simulink model "weightloss"  (R2022a)
settings: Solver=VariableStepAuto  StartTime=0.0  StopTime=500  RelTol=1e-3
libraries: cstblocks x1
settings Model: Creator=anthony  LastModifiedBy=anthony

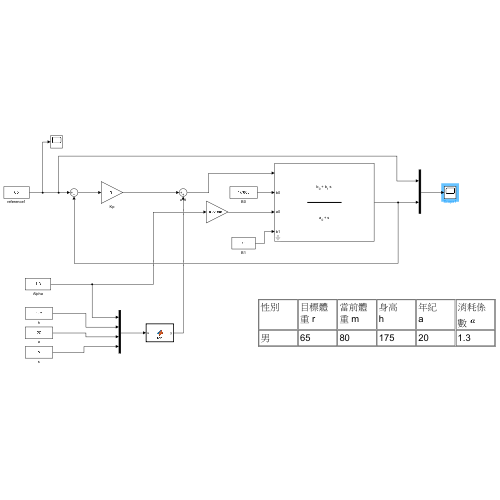
[thumbnail: Simulink's stored preview of the top-level diagram]
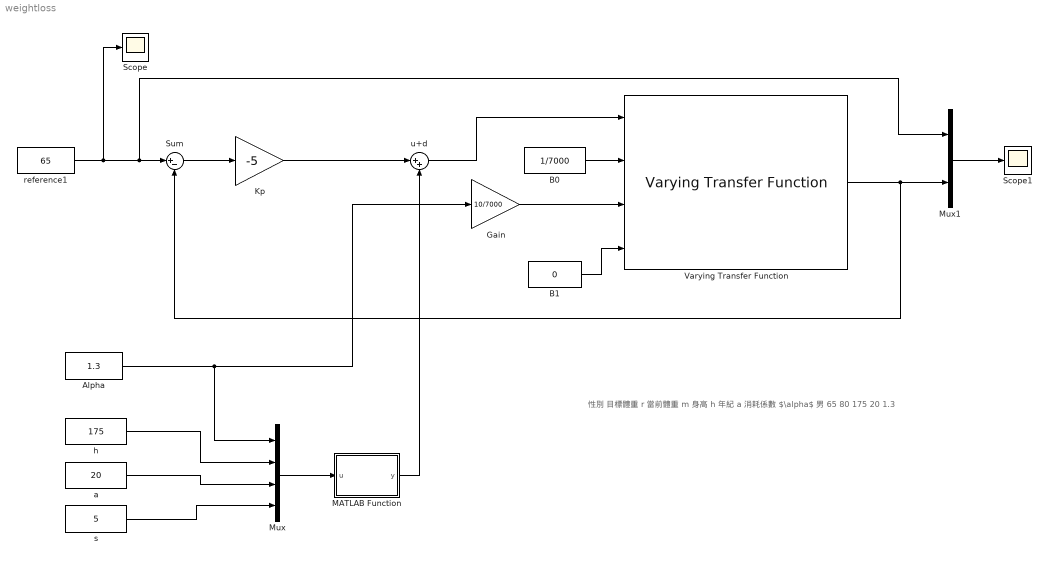
== system weightloss ==
  note: 性別
      | 目標體重 r
      | 當前體重 m
      | 身高
      | h
      | 年紀
      | a
      | 消耗係數 $\alpha$
      |
      | 男
      | 65
      | 80
      | 175
      | 20
      | 1.3
  Alpha : Constant  Value=1.3
  B0 : Constant  Value=1/7000
  B1 : Constant  Value=0
  Gain : Gain  Gain=10/7000
  Kp : Gain  Gain=-5
  MATLAB Function : MATLAB Function  TreatAsAtomicUnit=on
  Mux : Mux
  Mux1 : Mux  Inputs=2
  Scope : Scope
  Scope1 : Scope
  Sum : Sum  Inputs=|+-
  Varying Transfer Function : cstblocks/Linear Parameter Varying/Varying Transfer Function  N=1
      link override Integrator1: InitialCondition=80
  a : Constant  Value=20
  h : Constant  Value=175
  reference1 : Constant  Value=65
  s : Constant  Value=5
  u+d : Sum  Inputs=|++
  wires:
  Alpha/1 -> Mux/1, Gain/1
  Mux/1 -> MATLAB Function/1(u)
  Varying Transfer Function/1 -> Mux1/2, Sum/2
  B1/1 -> Varying Transfer Function/4
  Gain/1 -> Varying Transfer Function/3
  B0/1 -> Varying Transfer Function/2
  s/1 -> Mux/4
  a/1 -> Mux/3
  h/1 -> Mux/2
  Kp/1 -> u+d/1
  Sum/1 -> Kp/1
  MATLAB Function/1(y) -> u+d/2
  u+d/1 -> Varying Transfer Function/1
  reference1/1 -> Scope/1, Mux1/1, Sum/1
  Mux1/1 -> Scope1/1

== matlab function weightloss/MATLAB Function ==
  data: u input; y output
function y = fcn(u)
y = -u(1)*(6.25*u(2)-5*u(3)+u(4));
